simulink model "Simulator_hquad_lqri_traj"  (Simulink 7.8)
settings: Solver=ode3  StartTime=0.0  StopTime=40  FixedStep=Ts  RelTol=1e-3
values from neighbouring files (symbols this model uses):
  Ts = 0.02    [kostas_malakies.mat]    (also in kostas_malakies2.mat; main.m; main_last.m; matlab.mat = 0.08)
  Ts_slow = 0.02    [kostas_malakies.mat]    (also in kostas_malakies2.mat; main.m; main_last.m)
libraries: simulink x13, Hquad_control_LIB_LQRI x5, sdolib x4, Hqaud_model_LIB_SI x1
settings Model: Creator=andi  LastModifiedBy=burrimi
settings DebuggingCC: InheritedTsInSrcMsg=none  FcnCallInpInsideContextMsg=Use local settings  StrictBusMsg=Warning
settings SFSimCC: SimParseCustomCode=off

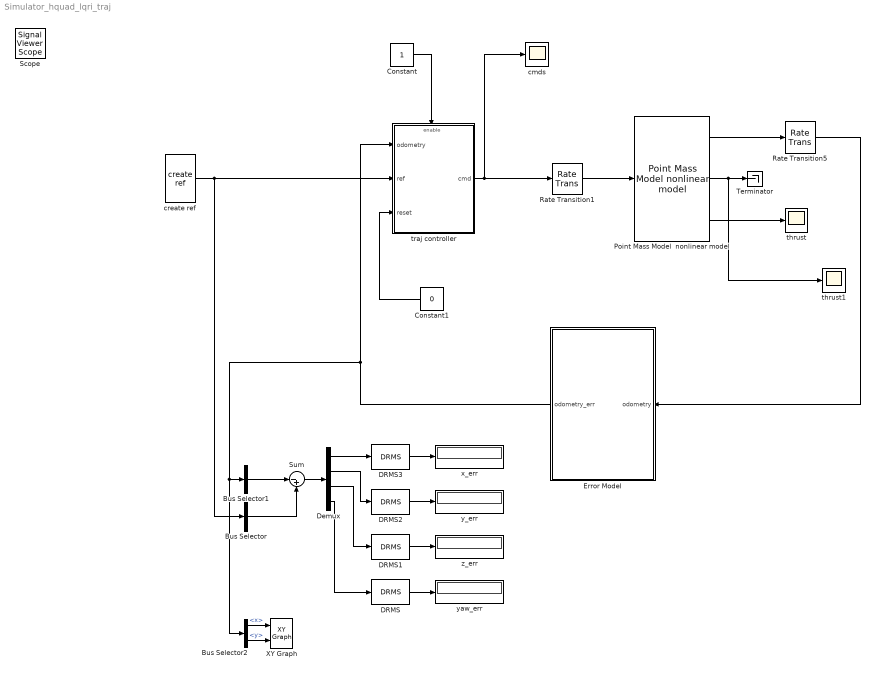
== system Simulator_hquad_lqri_traj ==
  Bus Selector : BusSelector  OutputSignals=pose_ref.x_ref,pose_ref.y_ref,pose_ref.z_ref,pose_ref.yaw_ref  OutputAsBus=on
  Bus Selector1 : BusSelector  OutputSignals=pos.x,pos.y,pos.z,rpy.yaw  OutputAsBus=on
  Bus Selector2 : BusSelector  OutputSignals=pos.x,pos.y
  Constant : Constant
  Constant1 : Constant  Value=0
  DRMS{,1..3} (4 alike) : sdolib/RMS Blocks/DRMS  Ts=Ts
  Demux : Demux
  Error Model : Subsystem
  Point Mass Model  nonlinear model : Hqaud_model_LIB_SI/Point Mass Model  nonlinear model
  Rate Transition1 : RateTransition  OutPortSampleTime=Ts
  Rate Transition5 : RateTransition  OutPortSampleTime=Ts
  Sum : Sum  Inputs=|-+
  Terminator : Terminator
  XY Graph : simulink/Sinks/XY Graph  xmin=-2  xmax=2  ymin=-2  ymax=2  st=-1
  cmds : Scope
      settings: TimeRange=40  YMin=-0.5  YMax=0.5
  create ref : Hquad_control_LIB_LQRI/create ref
  thrust : Scope
      settings: TimeRange=40  YMin=113.9130434782609  YMax=138.2608695652174  SaveName=ScopeData8
  thrust1 : Scope
      settings: TimeRange=40  YMin=-2  YMax=6  SaveName=ScopeData9
  traj controller : Subsystem  AncestorBlock=Hquad_control_LIB_LQRI/traj controller
  x_err : Display
  y_err : Display
  yaw_err : Display
  z_err : Display
  Scope : SignalViewerScope  IOType=viewer  LegendLocations="321.25       180.625         123.5       128.125"  RefreshTime=0.035000
      settings: ShowLegends=on
  wires:
  Point Mass Model  nonlinear model/3 -> thrust/1
  traj controller/1(cmd) -> cmds/1, Rate Transition1/1
  Constant/1 -> traj controller/Enable
  Point Mass Model  nonlinear model/2 -> Terminator/1, thrust1/1
  Constant1/1 -> traj controller/3(reset)
  create ref/1 -> Bus Selector/1, traj controller/2(ref)
  Point Mass Model  nonlinear model/1 -> Rate Transition5/1
  Error Model/1(odometry_err) -> traj controller/1(odometry), Bus Selector1/1, Bus Selector2/1
  Rate Transition5/1 -> Error Model/1(odometry)
  Bus Selector1/1 -> Sum/1
  Bus Selector/1 -> Sum/2
  Sum/1 -> Demux/1
  Demux/1 -> DRMS3/1
  Demux/2 -> DRMS2/1
  Demux/3 -> DRMS1/1
  Demux/4 -> DRMS/1
  DRMS/1 -> yaw_err/1
  DRMS1/1 -> z_err/1
  DRMS2/1 -> y_err/1
  DRMS3/1 -> x_err/1
  Rate Transition1/1 -> Point Mass Model  nonlinear model/1
  Bus Selector2/1 -> XY Graph/1  "<x>"
  Bus Selector2/2 -> XY Graph/2  "<y>"

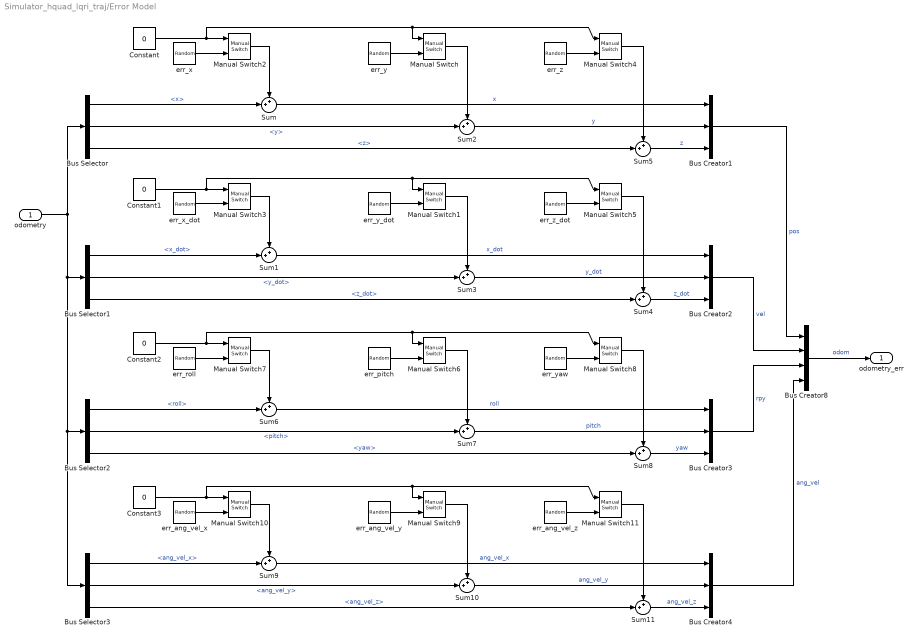
== system Simulator_hquad_lqri_traj/Error Model ==
  odometry : Inport
  Bus Creator{1..4} (4 alike) : BusCreator  Inputs=3
  Bus Creator8 : BusCreator
  Bus Selector : BusSelector  OutputSignals=pos.x,pos.y,pos.z
  Bus Selector1 : BusSelector  OutputSignals=vel.x_dot,vel.y_dot,vel.z_dot
  Bus Selector2 : BusSelector  OutputSignals=rpy.roll,rpy.pitch,rpy.yaw
  Bus Selector3 : BusSelector  OutputSignals=ang_vel.ang_vel_x,ang_vel.ang_vel_y,ang_vel.ang_vel_z
  Constant{,1..3} (4 alike) : Constant  Value=0
  Manual Switch{,1..11} (12 alike) : simulink/Signal Routing/Manual Switch  sw=1  action=0  varsize=off
  Sum{,1..11} (12 alike) : Sum  Inputs=++|  SampleTime=Ts_slow
  err_ang_vel_x : RandomNumber  Variance=0.0001  SampleTime=Ts_slow
  err_ang_vel_y : RandomNumber  Variance=0.0001  SampleTime=Ts_slow
  err_ang_vel_z : RandomNumber  Variance=0.0001  SampleTime=Ts_slow
  err_pitch : RandomNumber  Variance=0.0001  SampleTime=Ts_slow
  err_roll : RandomNumber  Variance=0.0001  SampleTime=Ts_slow
  err_x : RandomNumber  Variance=0.000707  SampleTime=Ts_slow
  err_x_dot : RandomNumber  Variance=0.0001  SampleTime=Ts_slow
  err_y : RandomNumber  Variance=0.000707  SampleTime=Ts_slow
  err_y_dot : RandomNumber  Variance=0.0001  SampleTime=Ts_slow
  err_yaw : RandomNumber  Variance=0.0001  SampleTime=Ts_slow
  err_z : RandomNumber  Variance=0.000707  SampleTime=Ts_slow
  err_z_dot : RandomNumber  Variance=0.0001  SampleTime=Ts_slow
  odometry_err : Outport
  wires:
  err_z/1 -> Manual Switch4/2
  Manual Switch4/1 -> Sum5/1
  err_y/1 -> Manual Switch/2
  Manual Switch/1 -> Sum2/1
  err_x/1 -> Manual Switch2/2
  Manual Switch2/1 -> Sum/1
  Sum/1 -> Bus Creator1/1  "x"
  Bus Creator1/1 -> Bus Creator8/1  "pos"
  Sum2/1 -> Bus Creator1/2  "y"
  Sum5/1 -> Bus Creator1/3  "z"
  odometry/1 -> Bus Selector/1, Bus Selector2/1, Bus Selector3/1, Bus Selector1/1
  Bus Selector/1 -> Sum/2  "<x>"
  Bus Selector/2 -> Sum2/2  "<y>"
  Bus Selector/3 -> Sum5/2  "<z>"
  Constant/1 -> Manual Switch2/1, Manual Switch/1, Manual Switch4/1
  err_z_dot/1 -> Manual Switch5/2
  Manual Switch5/1 -> Sum4/1
  err_y_dot/1 -> Manual Switch1/2
  Manual Switch1/1 -> Sum3/1
  err_x_dot/1 -> Manual Switch3/2
  Manual Switch3/1 -> Sum1/1
  Sum1/1 -> Bus Creator2/1  "x_dot"
  Sum3/1 -> Bus Creator2/2  "y_dot"
  Sum4/1 -> Bus Creator2/3  "z_dot"
  Bus Selector1/1 -> Sum1/2  "<x_dot>"
  Bus Selector1/2 -> Sum3/2  "<y_dot>"
  Bus Selector1/3 -> Sum4/2  "<z_dot>"
  Constant1/1 -> Manual Switch3/1, Manual Switch1/1, Manual Switch5/1
  Bus Creator2/1 -> Bus Creator8/2  "vel"
  err_yaw/1 -> Manual Switch8/2
  Manual Switch8/1 -> Sum8/1
  err_pitch/1 -> Manual Switch6/2
  Manual Switch6/1 -> Sum7/1
  err_roll/1 -> Manual Switch7/2
  Manual Switch7/1 -> Sum6/1
  Sum6/1 -> Bus Creator3/1  "roll"
  Sum7/1 -> Bus Creator3/2  "pitch"
  Sum8/1 -> Bus Creator3/3  "yaw"
  Bus Selector2/1 -> Sum6/2  "<roll>"
  Bus Selector2/2 -> Sum7/2  "<pitch>"
  Bus Selector2/3 -> Sum8/2  "<yaw>"
  Constant2/1 -> Manual Switch7/1, Manual Switch6/1, Manual Switch8/1
  Bus Creator3/1 -> Bus Creator8/3  "rpy"
  err_ang_vel_z/1 -> Manual Switch11/2
  Manual Switch11/1 -> Sum11/1
  err_ang_vel_y/1 -> Manual Switch9/2
  Manual Switch9/1 -> Sum10/1
  err_ang_vel_x/1 -> Manual Switch10/2
  Manual Switch10/1 -> Sum9/1
  Sum9/1 -> Bus Creator4/1  "ang_vel_x"
  Sum10/1 -> Bus Creator4/2  "ang_vel_y"
  Sum11/1 -> Bus Creator4/3  "ang_vel_z"
  Bus Selector3/1 -> Sum9/2  "<ang_vel_x>"
  Bus Selector3/2 -> Sum10/2  "<ang_vel_y>"
  Bus Selector3/3 -> Sum11/2  "<ang_vel_z>"
  Constant3/1 -> Manual Switch10/1, Manual Switch9/1, Manual Switch11/1
  Bus Creator4/1 -> Bus Creator8/4  "ang_vel"
  Bus Creator8/1 -> odometry_err/1  "odom"

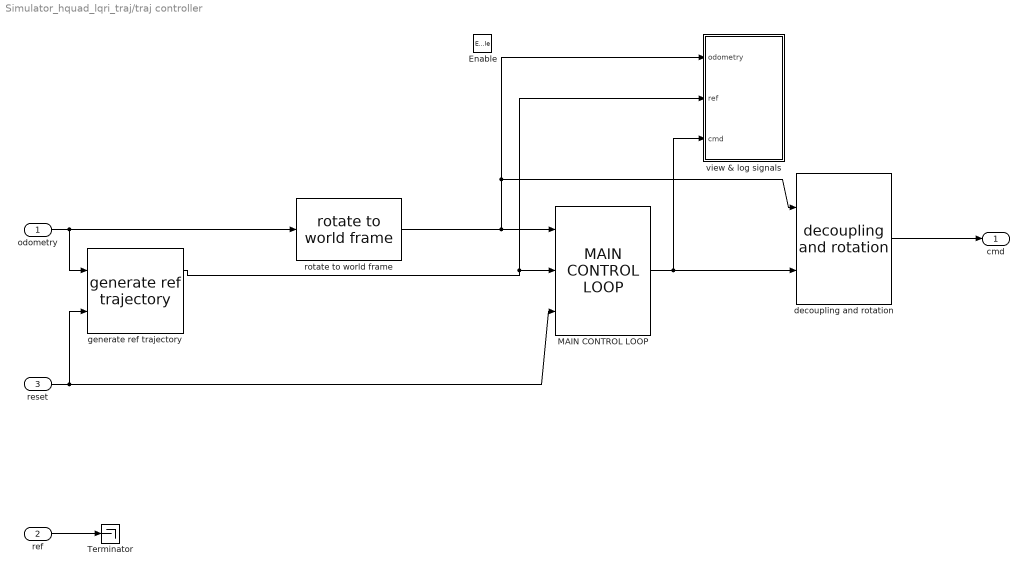
== system Simulator_hquad_lqri_traj/traj controller ==
  odometry : Inport
  ref : Inport  Port=2
  reset : Inport  Port=3
  Enable : EnablePort  StatesWhenEnabling=reset
  MAIN CONTROL LOOP : Hquad_control_LIB_LQRI/MAIN CONTROL LOOP
  Terminator : Terminator
  decoupling and rotation : Hquad_control_LIB_LQRI/decoupling and rotation  Priority=3
  generate ref trajectory : Hquad_control_LIB_LQRI/generate ref trajectory
  rotate to world frame : Hquad_control_LIB_LQRI/rotate to world frame  Priority=1
  view & log signals : Subsystem  AncestorBlock=Hquad_control_LIB_LQRI/view & log signals
  cmd : Outport
  wires:
  decoupling and rotation/1 -> cmd/1
  MAIN CONTROL LOOP/1 -> decoupling and rotation/2, view & log signals/3(cmd)
  rotate to world frame/1 -> MAIN CONTROL LOOP/1, decoupling and rotation/1, view & log signals/1(odometry)
  odometry/1 -> rotate to world frame/1, generate ref trajectory/1
  ref/1 -> Terminator/1
  reset/1 -> MAIN CONTROL LOOP/3, generate ref trajectory/2
  generate ref trajectory/1 -> view & log signals/2(ref), MAIN CONTROL LOOP/2

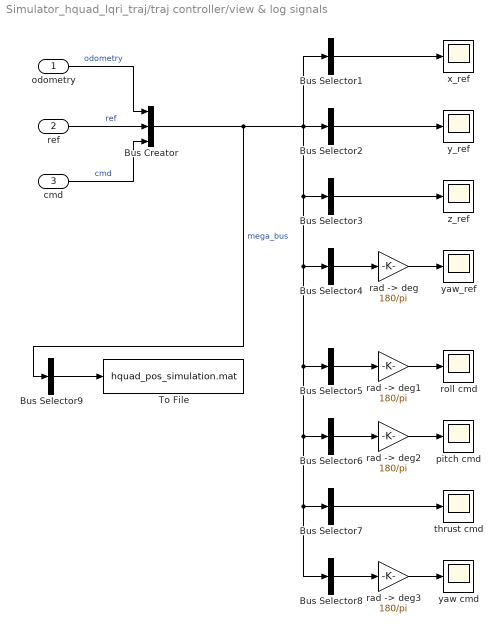
== system Simulator_hquad_lqri_traj/traj controller/view & log signals ==
  odometry : Inport
  ref : Inport  Port=2
  cmd : Inport  Port=3
  Bus Creator : BusCreator  Inputs=3
  Bus Selector1 : BusSelector  OutputSignals=odometry.pos.x,odometry.vel.x_dot,ref.pose_ref.x_ref,ref.vel_ref.x_dot_ref  OutputAsBus=on
  Bus Selector2 : BusSelector  OutputSignals=odometry.pos.y,odometry.vel.y_dot,ref.pose_ref.y_ref,ref.vel_ref.y_dot_ref  OutputAsBus=on
  Bus Selector3 : BusSelector  OutputSignals=odometry.pos.z,odometry.vel.z_dot,ref.pose_ref.z_ref,ref.vel_ref.z_dot_ref  OutputAsBus=on
  Bus Selector4 : BusSelector  OutputSignals=odometry.rpy.yaw,odometry.ang_vel.ang_vel_z,ref.pose_ref.yaw_ref,ref.vel_ref.yaw_dot_ref  OutputAsBus=on
  Bus Selector5 : BusSelector  OutputSignals=odometry.rpy.roll,odometry.ang_vel.ang_vel_x,cmd.roll_cmd  OutputAsBus=on
  Bus Selector6 : BusSelector  OutputSignals=odometry.rpy.pitch,odometry.ang_vel.ang_vel_y,cmd.pitch_cmd  OutputAsBus=on
  Bus Selector7 : BusSelector  OutputSignals=odometry.pos.z,ref.pose_ref.z_ref,cmd.thrust_cmd  OutputAsBus=on
  Bus Selector8 : BusSelector  OutputSignals=odometry.rpy.yaw,odometry.ang_vel.ang_vel_z,cmd.yaw_rate_cmd  OutputAsBus=on
  Bus Selector9 : BusSelector  OutputSignals=odometry.pos.x,odometry.vel.x_dot,odometry.rpy.pitch,ref.pose_ref.x_ref,cmd.pitch_cmd,odometry.pos.y,odometry.vel.y_dot,odometry.rpy.roll,ref.pose_ref.y_ref,cmd.roll_cmd,odometry.pos.z,odometry.vel.z_dot,ref.pose_ref.z_ref,cmd.thrust_cmd,odometry.rpy.yaw,odometry.ang_vel.ang_vel_z,ref.pose_ref.yaw_ref,cmd.yaw_rate_cmd  OutputAsBus=on
  To File : ToFile  Filename=hquad_pos_simulation.mat  MatrixName=hquad_pos_simulation
  pitch cmd : Scope
      settings: YMin=-15  YMax=15  SaveName=ScopeData2
  rad -> deg{,1..3} (4 alike) : Gain  Gain=180/pi
  roll cmd : Scope
      settings: YMin=-100  YMax=100
  thrust cmd : Scope
      settings: YMin=-3  YMax=3  SaveName=ScopeData11
  x_ref : Scope
      settings: TimeRange=40  YMin=-1.5  YMax=1.5  SaveName=ScopeData3
  y_ref : Scope
      settings: TimeRange=40  YMin=-1.5  YMax=1.5
  yaw cmd : Scope
      settings: YMin=-60  YMax=-0  SaveName=ScopeData10
  yaw_ref : Scope
      settings: TimeRange=39.996  YMin=0  YMax=3250  SaveName=ScopeData8
  z_ref : Scope
      settings: YMin=-0.05  YMax=1.05  SaveName=ScopeData5
  wires:
  Bus Selector9/1 -> To File/1
  "rad -> deg"/1 -> yaw_ref/1
  "rad -> deg1"/1 -> roll cmd/1
  "rad -> deg2"/1 -> pitch cmd/1
  "rad -> deg3"/1 -> yaw cmd/1
  odometry/1 -> Bus Creator/1  "odometry"
  ref/1 -> Bus Creator/2  "ref"
  cmd/1 -> Bus Creator/3  "cmd"
  Bus Creator/1 -> Bus Selector9/1, Bus Selector1/1, Bus Selector2/1, Bus Selector3/1, Bus Selector4/1, Bus Selector5/1, Bus Selector6/1, Bus Selector7/1, Bus Selector8/1  "mega_bus"
  Bus Selector1/1 -> x_ref/1
  Bus Selector2/1 -> y_ref/1
  Bus Selector3/1 -> z_ref/1
  Bus Selector4/1 -> "rad -> deg"/1
  Bus Selector7/1 -> thrust cmd/1
  Bus Selector5/1 -> "rad -> deg1"/1
  Bus Selector6/1 -> "rad -> deg2"/1
  Bus Selector8/1 -> "rad -> deg3"/1
